simulink model "SF102A_MotCtrlPrmEstimn"  (R2013b)
settings: Solver=FixedStepDiscrete  StartTime=0.0  StopTime=1  FixedStep=0.002  RelTol=1e-3
values from neighbouring files (symbols this model uses):
  MotCtrlPrmEstimnFetRNom = DataDict.Calibration    [SF102A_MotCtrlPrmEstimn_DataDict.m]
  MotCtrlPrmEstimnFetThermCoeff = DataDict.Calibration    [SF102A_MotCtrlPrmEstimn_DataDict.m]
  MotCtrlPrmEstimnMagThermCoeff = DataDict.Calibration    [SF102A_MotCtrlPrmEstimn_DataDict.m]
  MotCtrlPrmEstimnMotBackEmfConNom = DataDict.Calibration    [SF102A_MotCtrlPrmEstimn_DataDict.m]
  MotCtrlPrmEstimnMotBackEmfConSatnScaIvtrLoaMtgtn = DataDict.Calibration    [SF102A_MotCtrlPrmEstimn_DataDict.m]
  MotCtrlPrmEstimnMotInduDaxIvtrLoaMtgtn = DataDict.Calibration    [SF102A_MotCtrlPrmEstimn_DataDict.m]
  MotCtrlPrmEstimnMotInduDaxNom = DataDict.Calibration    [SF102A_MotCtrlPrmEstimn_DataDict.m]
  MotCtrlPrmEstimnMotInduQaxIvtrLoaMtgtn = DataDict.Calibration    [SF102A_MotCtrlPrmEstimn_DataDict.m]
  MotCtrlPrmEstimnMotInduQaxNom = DataDict.Calibration    [SF102A_MotCtrlPrmEstimn_DataDict.m]
  MotCtrlPrmEstimnMotRNom = DataDict.Calibration    [SF102A_MotCtrlPrmEstimn_DataDict.m]
  MotCtrlPrmEstimnMotWidgThermCoeff = DataDict.Calibration    [SF102A_MotCtrlPrmEstimn_DataDict.m]
  MotCtrlPrmEstimnTNom = DataDict.Calibration    [SF102A_MotCtrlPrmEstimn_DataDict.m]
libraries: NxtrLim x12, NxtrNvM x3, FixdToFloat x3, FloatToFixd x2, BilnrIntrpnCmnX x2, simulink x1, LnrIntrpn x1
(part 2 of 2)

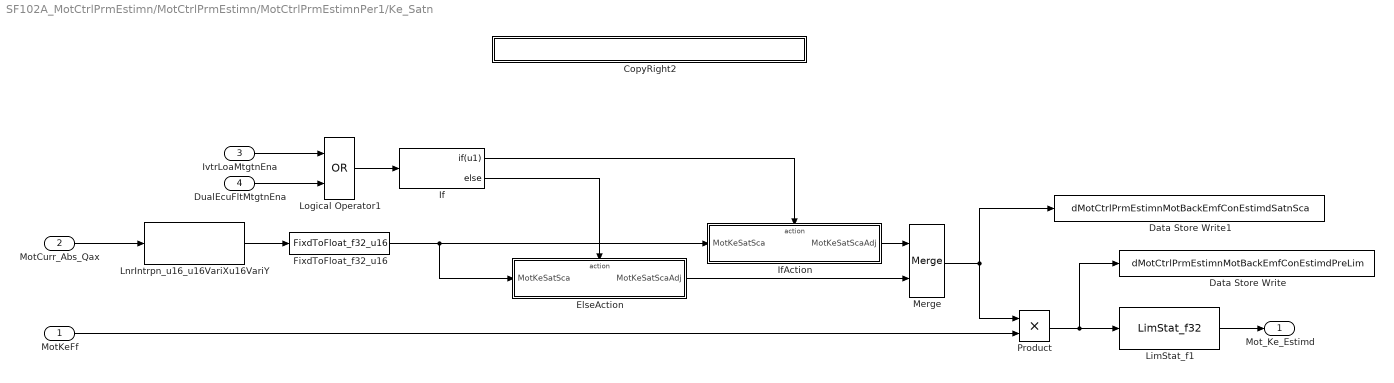
== system SF102A_MotCtrlPrmEstimn/MotCtrlPrmEstimn/MotCtrlPrmEstimnPer1/Ke_Satn ==
  MotKeFf : Inport  RequirementInfo="{'linktype_rmi_doors' '0000bb41 (/E-STEER Core/SubSystem Specifications/Application Functions/SF99/SF102A Motor Control Parameter Estimation)' '#SF102A_51' 'true' 'REQ:  SF102A_51' '' } %GIDa_ca68ec69_3fc5_4f7c_b88c_595812cbfbcb"
  MotCurr_Abs_Qax : Inport  RequirementInfo="{'linktype_rmi_doors' '0000bb41 (/E-STEER Core/SubSystem Specifications/Application Functions/SF99/SF102A Motor Control Parameter Estimation)' '#SF102A_50' 'true' 'REQ:  SF102A_50' '' ; 'linktype_rmi_doors' '0000bb41 (/E-STEER Core/SubSystem Specifications/Application Functions/SF99/SF102A Motor Control Parameter Estimation)' '#SF102A_51' 'true' 'REQ:  SF102A_51' '' } %GIDa_2c278c4c_34d3_4811_86bc_36d03b3a96ac"  Port=2
  IvtrLoaMtgtnEna : Inport  RequirementInfo={} %GIDa_55b474c1_2280_46dc_85c4_036e6c47f197  Port=3
  DualEcuFltMtgtnEna : Inport  RequirementInfo={} %GIDa_d4aecfc1_0bde_4cba_a1f2_c868140dd92f  Port=4
  CopyRight2 : Subsystem  Description=|  mask(Copyright Information){none=on}
      | Copyright info block.                                               
      |                                                                     
      | Place copyright information at the top of every subsystem in design.
      mask prompts: none "No parameters"
      mask help: Place copyright information at the top of every subsystem in design.
      mask Display:
      | NxtrConf = 'Nexteer Confidential';
      | 
      | sys = bdroot; %handle for the current model ("system")
      | first = get_param(sys,'Created');
      | if(isempty(first))
      |     first = datestr(now,'yyyy');
      | else
      |     first = first(end-3:end);  %year is last four digits
      | end
      | 
      | last = get_param(sys,'LastModifiedDate');
      | if isempty(last)
      |     last = datestr(now,'yyyy');
      | else
      |     last = last(end-3:end);
      | end
      | 
      | if strcmp(first,last)
      |     fprintf('%s -- Copyright %s Nexteer',NxtrConf,first)
      | else
      |     fprintf('%s -- %s%s- %s Nexteer',NxtrConf,char(169),first,last)
      | end
  Data Store Write : DataStoreWrite  DataStoreName=dMotCtrlPrmEstimnMotBackEmfConEstimdPreLim
  Data Store Write1 : DataStoreWrite  DataStoreName=dMotCtrlPrmEstimnMotBackEmfConEstimdSatnSca
  ElseAction : Subsystem  RequirementInfo={'linktype_rmi_doors' '0000bb41 (/E-STEER Core/SubSystem Specifications/Application Functions/SF99/SF102A Motor Control Parameter Estimation)' '#SF102A_98' 'true' 'REQ:SF102A_98' '' } %GIDa_66276068_9c00_412a_ba6b_6416dc8d8b98  TreatAsAtomicUnit=on
  FixdToFloat_f32_u16 : FixdToFloat/FixdToFloat_f32_u16  RequirementInfo="{'linktype_rmi_doors' '0000bb41 (/E-STEER Core/SubSystem Specifications/Application Functions/SF99/SF102A Motor Control Parameter Estimation)' '#SF102A_50' 'true' 'REQ:  SF102A_50' '' ; 'linktype_rmi_doors' '0000bb41 (/E-STEER Core/SubSystem Specifications/Application Functions/SF99/SF102A Motor Control Parameter Estimation)' '#SF102A_51' 'true' 'REQ:  SF102A_51' '' } %GIDa_30ff50c8_3b22_4b0c_a269_05ad7e058210"  Param1=14
  If : If  RequirementInfo={'linktype_rmi_doors' '0000bb41 (/E-STEER Core/SubSystem Specifications/Application Functions/SF99/SF102A Motor Control Parameter Estimation)' '#SF102A_98' 'true' 'REQ:SF102A_98' '' } %GIDa_a3456abc_87ca_4b4f_a759_32778ebeb971  IfExpression=u1
  IfAction : Subsystem  RequirementInfo={'linktype_rmi_doors' '0000bb41 (/E-STEER Core/SubSystem Specifications/Application Functions/SF99/SF102A Motor Control Parameter Estimation)' '#SF102A_98' 'true' 'REQ:SF102A_98' '' } %GIDa_37ca894a_f849_476d_86bb_7b83343cfe71  TreatAsAtomicUnit=on
      settings: RTWSystemCode=Inline
  LimStat_f1 : NxtrLim/LimStat_f32  RequirementInfo="{'linktype_rmi_doors' '0000bb41 (/E-STEER Core/SubSystem Specifications/Application Functions/SF99/SF102A Motor Control Parameter Estimation)' '#SF102A_58' 'true' 'REQ:  SF102A_58' '' ; 'linktype_rmi_doors' '0000bb41 (/E-STEER Core/SubSystem Specifications/Application Functions/SF99/SF102A Motor Control Parameter Estimation)' '#SF102A_77' 'true' 'REQ:  SF102A_77' '' } %GIDa_efba97fb_19df_4fbb_835b_1b2e4b8dafc6"  LoLim=MotCtrlPrmEstimnMotBackEmfConLoLim  HiLim=MotCtrlPrmEstimnMotBackEmfConHiLim
      settings: AttributesFormatString=|
      | Low Limit: %<LoLim>
      | High Limit:%<HiLim>
  LnrIntrpn_u16_u16VariXu16VariY : LnrIntrpn/LnrIntrpn_u16_u16VariXu16VariY  RequirementInfo="{'linktype_rmi_doors' '0000bb41 (/E-STEER Core/SubSystem Specifications/Application Functions/SF99/SF102A Motor Control Parameter Estimation)' '#SF102A_50' 'true' 'REQ:  SF102A_50' '' ; 'linktype_rmi_doors' '0000bb41 (/E-STEER Core/SubSystem Specifications/Application Functions/SF99/SF102A Motor Control Parameter Estimation)' '#SF102A_51' 'true' 'REQ:  SF102A_51' '' } %GIDa_d0625b03_476d_4e45_a255_0ebee113fbee"  XTbl=MotCtrlPrmEstimnMotBackEmfConSatnX  YTbl=MotCtrlPrmEstimnMotBackEmfConSatnY
      settings: AttributesFormatString=Lnr ( u16VariX , u16VariY )
  Logical Operator1 : Logic  Operator=OR  AllPortsSameDT=off  OutDataTypeStr=boolean
  Merge : Merge  RequirementInfo={'linktype_rmi_doors' '0000bb41 (/E-STEER Core/SubSystem Specifications/Application Functions/SF99/SF102A Motor Control Parameter Estimation)' '#SF102A_98' 'true' 'REQ:SF102A_98' '' } %GIDa_a953d2b4_b957_47a9_9e6b_14a5c79d3b44
  Product : Product  RequirementInfo="{'linktype_rmi_doors' '0000bb41 (/E-STEER Core/SubSystem Specifications/Application Functions/SF99/SF102A Motor Control Parameter Estimation)' '#SF102A_51' 'true' 'REQ:  SF102A_51' '' } %GIDa_5f6ae74a_60fe_41e9_b3da_6065efd4cb7b"
  Mot_Ke_Estimd : Outport  RequirementInfo="{'linktype_rmi_doors' '0000bb41 (/E-STEER Core/SubSystem Specifications/Application Functions/SF99/SF102A Motor Control Parameter Estimation)' '#SF102A_51' 'true' 'REQ:  SF102A_51' '' } %GIDa_09a11d9d_3369_4bbb_9775_2492efeb312e"
  wires:
  LnrIntrpn_u16_u16VariXu16VariY/1 -> FixdToFloat_f32_u16/1
  MotKeFf/1 -> Product/2
  Product/1 -> Data Store Write/1, LimStat_f1/1
  LimStat_f1/1 -> Mot_Ke_Estimd/1
  Merge/1 -> Product/1, Data Store Write1/1
  MotCurr_Abs_Qax/1 -> LnrIntrpn_u16_u16VariXu16VariY/1
  If/2 -> ElseAction/Action
  If/1 -> IfAction/Action
  ElseAction/1(MotKeSatScaAdj) -> Merge/2
  IfAction/1(MotKeSatScaAdj) -> Merge/1
  FixdToFloat_f32_u16/1 -> ElseAction/1(MotKeSatSca), IfAction/1(MotKeSatSca)
  IvtrLoaMtgtnEna/1 -> Logical Operator1/1
  DualEcuFltMtgtnEna/1 -> Logical Operator1/2
  Logical Operator1/1 -> If/1

== system SF102A_MotCtrlPrmEstimn/MotCtrlPrmEstimn/MotCtrlPrmEstimnPer2/CopyRight2 ==

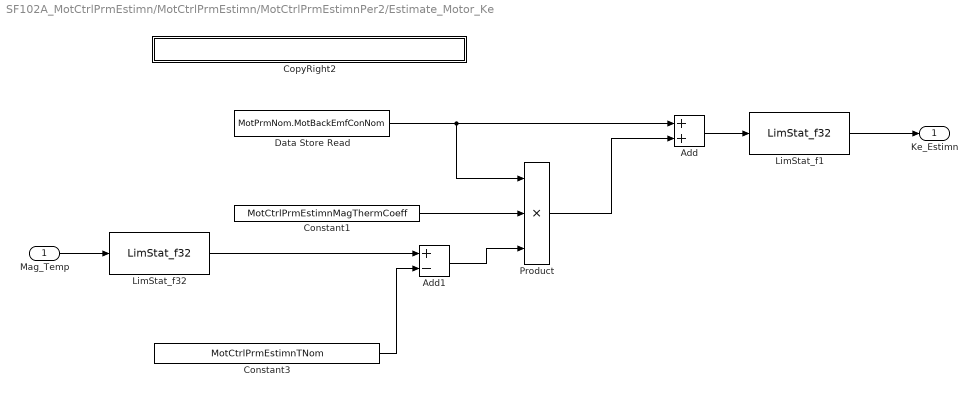
== system SF102A_MotCtrlPrmEstimn/MotCtrlPrmEstimn/MotCtrlPrmEstimnPer2/Estimate_Motor_Ke ==
  Mag_Temp : Inport  RequirementInfo="{'linktype_rmi_doors' '0000bb41 (/E-STEER Core/SubSystem Specifications/Application Functions/SF99/SF102A Motor Control Parameter Estimation)' '#SF102A_79' 'true' 'REQ:  SF102A_79' '' } %GIDa_27ec31af_a9b0_49cc_af07_57667b1f493e"
  Add : Sum  RequirementInfo="{'linktype_rmi_doors' '0000bb41 (/E-STEER Core/SubSystem Specifications/Application Functions/SF99/SF102A Motor Control Parameter Estimation)' '#SF102A_79' 'true' 'REQ:  SF102A_79' '' } %GIDa_032c7cc2_7709_47c2_b088_cd2d10e989b2"
  Add1 : Sum  RequirementInfo="{'linktype_rmi_doors' '0000bb41 (/E-STEER Core/SubSystem Specifications/Application Functions/SF99/SF102A Motor Control Parameter Estimation)' '#SF102A_79' 'true' 'REQ:  SF102A_79' '' } %GIDa_325acd5b_255d_4854_912c_df54e826c433"  Inputs=+-
  Constant1 : Constant  RequirementInfo="{'linktype_rmi_doors' '0000bb41 (/E-STEER Core/SubSystem Specifications/Application Functions/SF99/SF102A Motor Control Parameter Estimation)' '#SF102A_79' 'true' 'REQ:  SF102A_79' '' } %GIDa_95a68016_cdb7_4865_bd2d_230faec756a9"  Value=MotCtrlPrmEstimnMagThermCoeff
  Constant3 : Constant  RequirementInfo="{'linktype_rmi_doors' '0000bb41 (/E-STEER Core/SubSystem Specifications/Application Functions/SF99/SF102A Motor Control Parameter Estimation)' '#SF102A_79' 'true' 'REQ:  SF102A_79' '' } %GIDa_62d1b4b8_0c50_4cfb_896c_98b14855d1cc"  Value=MotCtrlPrmEstimnTNom
  CopyRight2 : Subsystem  Description=|  mask(Copyright Information){none=on}
      | Copyright info block.                                               
      |                                                                     
      | Place copyright information at the top of every subsystem in design.
      mask prompts: none "No parameters"
      mask help: Place copyright information at the top of every subsystem in design.
      mask Display:
      | NxtrConf = 'Nexteer Confidential';
      | 
      | sys = bdroot; %handle for the current model ("system")
      | first = get_param(sys,'Created');
      | if(isempty(first))
      |     first = datestr(now,'yyyy');
      | else
      |     first = first(end-3:end);  %year is last four digits
      | end
      | 
      | last = get_param(sys,'LastModifiedDate');
      | if isempty(last)
      |     last = datestr(now,'yyyy');
      | else
      |     last = last(end-3:end);
      | end
      | 
      | if strcmp(first,last)
      |     fprintf('%s -- Copyright %s Nexteer',NxtrConf,first)
      | else
      |     fprintf('%s -- %s%s- %s Nexteer',NxtrConf,char(169),first,last)
      | end
  Data Store Read : DataStoreRead  RequirementInfo="{'linktype_rmi_doors' '0000bb41 (/E-STEER Core/SubSystem Specifications/Application Functions/SF99/SF102A Motor Control Parameter Estimation)' '#SF102A_79' 'true' 'REQ:  SF102A_79' '' } %GIDa_645f74b9_1f8d_46ad_9bf2_de69bb92e4a8"  DataStoreName=MotPrmNom  DataStoreElements=MotPrmNom.MotBackEmfConNom
  LimStat_f1 : NxtrLim/LimStat_f32  RequirementInfo="{'linktype_rmi_doors' '0000bb41 (/E-STEER Core/SubSystem Specifications/Application Functions/SF99/SF102A Motor Control Parameter Estimation)' '#SF102A_58' 'true' 'REQ:  SF102A_58' '' ; 'linktype_rmi_doors' '0000bb41 (/E-STEER Core/SubSystem Specifications/Application Functions/SF99/SF102A Motor Control Parameter Estimation)' '#SF102A_77' 'true' 'REQ:  SF102A_77' '' } %GIDa_eaf1ef11_d061_4c62_ac0d_c6cc858486f6"  LoLim=MotCtrlPrmEstimnMotBackEmfConLoLim  HiLim=MotCtrlPrmEstimnMotBackEmfConHiLim
      settings: AttributesFormatString=|
      | Low Limit: %<LoLim>
      | High Limit:%<HiLim>
  LimStat_f32 : NxtrLim/LimStat_f32  RequirementInfo="{'linktype_rmi_doors' '0000bb41 (/E-STEER Core/SubSystem Specifications/Application Functions/SF99/SF102A Motor Control Parameter Estimation)' '#SF102A_79' 'true' 'REQ:  SF102A_79' '' ; 'linktype_rmi_doors' '0000bb41 (/E-STEER Core/SubSystem Specifications/Application Functions/SF99/SF102A Motor Control Parameter Estimation)' '#SF102A_77' 'true' 'REQ:  SF102A_77' '' ; 'linktype_rmi_doors' '0000bb41 (/E-STEER Core/SubSystem Specifications/Application Functions/SF99/SF102A Motor Control Parameter Estimation)' '#SF102A_78' 'true' 'REQ:  SF102A_78' '' } %GIDa_c2f1950b_3da8_40ec_be6a_a30c98ab318e"  LoLim=MAGNETTESTLOLIM_DEGCGRD_F32  HiLim=MAGNETTESTHILIM_DEGCGRD_F32
      settings: AttributesFormatString=|
      | Low Limit: %<LoLim>
      | High Limit:%<HiLim>
  Product : Product  RequirementInfo="{'linktype_rmi_doors' '0000bb41 (/E-STEER Core/SubSystem Specifications/Application Functions/SF99/SF102A Motor Control Parameter Estimation)' '#SF102A_79' 'true' 'REQ:  SF102A_79' '' } %GIDa_beae5c53_6cdc_4a5b_91cf_3f5121611092"  Inputs=3
  Ke_Estimn : Outport  RequirementInfo="{'linktype_rmi_doors' '0000bb41 (/E-STEER Core/SubSystem Specifications/Application Functions/SF99/SF102A Motor Control Parameter Estimation)' '#SF102A_79' 'true' 'REQ:  SF102A_79' '' } %GIDa_fc83a985_17ec_4189_8e4e_4c54ef9d1b52"
  wires:
  Data Store Read/1 -> Add/1, Product/1
  Mag_Temp/1 -> LimStat_f32/1
  Constant3/1 -> Add1/2
  Add1/1 -> Product/3
  Constant1/1 -> Product/2
  Product/1 -> Add/2
  LimStat_f32/1 -> Add1/1
  Add/1 -> LimStat_f1/1
  LimStat_f1/1 -> Ke_Estimn/1

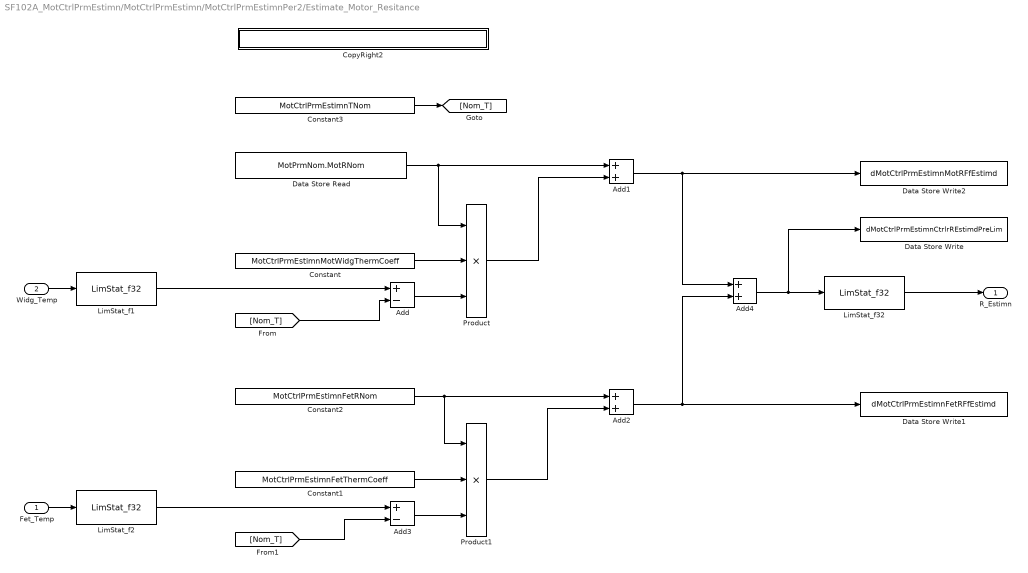
== system SF102A_MotCtrlPrmEstimn/MotCtrlPrmEstimn/MotCtrlPrmEstimnPer2/Estimate_Motor_Resitance ==
  Fet_Temp : Inport  RequirementInfo="{'linktype_rmi_doors' '0000bb41 (/E-STEER Core/SubSystem Specifications/Application Functions/SF99/SF102A Motor Control Parameter Estimation)' '#SF102A_79' 'true' 'REQ:  SF102A_79' '' } %GIDa_71261e82_d55a_46e2_88a5_a0108b8fb2d0"
  Widg_Temp : Inport  RequirementInfo="{'linktype_rmi_doors' '0000bb41 (/E-STEER Core/SubSystem Specifications/Application Functions/SF99/SF102A Motor Control Parameter Estimation)' '#SF102A_79' 'true' 'REQ:  SF102A_79' '' } %GIDa_114d5c54_a76c_45b6_89e5_6083f63a86c5"  Port=2
  Add : Sum  RequirementInfo="{'linktype_rmi_doors' '0000bb41 (/E-STEER Core/SubSystem Specifications/Application Functions/SF99/SF102A Motor Control Parameter Estimation)' '#SF102A_79' 'true' 'REQ:  SF102A_79' '' } %GIDa_9b0531e8_817d_417f_b08e_d44cb601da31"  Inputs=+-
  Add1 : Sum  RequirementInfo="{'linktype_rmi_doors' '0000bb41 (/E-STEER Core/SubSystem Specifications/Application Functions/SF99/SF102A Motor Control Parameter Estimation)' '#SF102A_79' 'true' 'REQ:  SF102A_79' '' } %GIDa_233736cd_2ef7_40b2_bc6f_cb61d0fd07dc"
  Add2 : Sum  RequirementInfo="{'linktype_rmi_doors' '0000bb41 (/E-STEER Core/SubSystem Specifications/Application Functions/SF99/SF102A Motor Control Parameter Estimation)' '#SF102A_79' 'true' 'REQ:  SF102A_79' '' } %GIDa_91af04b1_221a_42c8_9042_f241f3590e10"
  Add3 : Sum  RequirementInfo="{'linktype_rmi_doors' '0000bb41 (/E-STEER Core/SubSystem Specifications/Application Functions/SF99/SF102A Motor Control Parameter Estimation)' '#SF102A_79' 'true' 'REQ:  SF102A_79' '' } %GIDa_3a49abd4_5a0a_43ef_a101_a021352c1f05"  Inputs=+-
  Add4 : Sum  RequirementInfo="{'linktype_rmi_doors' '0000bb41 (/E-STEER Core/SubSystem Specifications/Application Functions/SF99/SF102A Motor Control Parameter Estimation)' '#SF102A_79' 'true' 'REQ:  SF102A_79' '' ; 'linktype_rmi_doors' '0000bb41 (/E-STEER Core/SubSystem Specifications/Application Functions/SF99/SF102A Motor Control Parameter Estimation)' '#SF102A_80' 'true' 'REQ:  SF102A_80' '' } %GIDa_9a8c8a44_bb52_4b56_826d_532e182878d7"
  Constant : Constant  RequirementInfo="{'linktype_rmi_doors' '0000bb41 (/E-STEER Core/SubSystem Specifications/Application Functions/SF99/SF102A Motor Control Parameter Estimation)' '#SF102A_79' 'true' 'REQ:  SF102A_79' '' } %GIDa_9b025c1a_f7a9_4777_8ff0_3314b9890bfc"  Value=MotCtrlPrmEstimnMotWidgThermCoeff
  Constant1 : Constant  RequirementInfo="{'linktype_rmi_doors' '0000bb41 (/E-STEER Core/SubSystem Specifications/Application Functions/SF99/SF102A Motor Control Parameter Estimation)' '#SF102A_79' 'true' 'REQ:  SF102A_79' '' } %GIDa_6745513d_e9f0_42ff_93c4_399939918044"  Value=MotCtrlPrmEstimnFetThermCoeff
  Constant2 : Constant  RequirementInfo="{'linktype_rmi_doors' '0000bb41 (/E-STEER Core/SubSystem Specifications/Application Functions/SF99/SF102A Motor Control Parameter Estimation)' '#SF102A_79' 'true' 'REQ:  SF102A_79' '' } %GIDa_eba00650_623e_448f_ba0b_e87ab14d84b4"  Value=MotCtrlPrmEstimnFetRNom
  Constant3 : Constant  RequirementInfo="{'linktype_rmi_doors' '0000bb41 (/E-STEER Core/SubSystem Specifications/Application Functions/SF99/SF102A Motor Control Parameter Estimation)' '#SF102A_79' 'true' 'REQ:  SF102A_79' '' } %GIDa_0212b6ce_dff5_41d0_8898_d0ec0ff62430"  Value=MotCtrlPrmEstimnTNom
  CopyRight2 : Subsystem  Description=|  mask(Copyright Information){none=on}
      | Copyright info block.                                               
      |                                                                     
      | Place copyright information at the top of every subsystem in design.
      mask prompts: none "No parameters"
      mask help: Place copyright information at the top of every subsystem in design.
      mask Display:
      | NxtrConf = 'Nexteer Confidential';
      | 
      | sys = bdroot; %handle for the current model ("system")
      | first = get_param(sys,'Created');
      | if(isempty(first))
      |     first = datestr(now,'yyyy');
      | else
      |     first = first(end-3:end);  %year is last four digits
      | end
      | 
      | last = get_param(sys,'LastModifiedDate');
      | if isempty(last)
      |     last = datestr(now,'yyyy');
      | else
      |     last = last(end-3:end);
      | end
      | 
      | if strcmp(first,last)
      |     fprintf('%s -- Copyright %s Nexteer',NxtrConf,first)
      | else
      |     fprintf('%s -- %s%s- %s Nexteer',NxtrConf,char(169),first,last)
      | end
  Data Store Read : DataStoreRead  RequirementInfo="{'linktype_rmi_doors' '0000bb41 (/E-STEER Core/SubSystem Specifications/Application Functions/SF99/SF102A Motor Control Parameter Estimation)' '#SF102A_79' 'true' 'REQ:  SF102A_79' '' } %GIDa_7acda2c8_c589_429d_b3c9_76fb565b8f54"  DataStoreName=MotPrmNom  DataStoreElements=MotPrmNom.MotRNom
  Data Store Write : DataStoreWrite  RequirementInfo="{'linktype_rmi_doors' '0000bb41 (/E-STEER Core/SubSystem Specifications/Application Functions/SF99/SF102A Motor Control Parameter Estimation)' '#SF102A_79' 'true' 'REQ:  SF102A_79' '' } %GIDa_bc42402b_ab84_4d6d_9d03_69266616b3e8"  DataStoreName=dMotCtrlPrmEstimnCtrlrREstimdPreLim
  Data Store Write1 : DataStoreWrite  RequirementInfo="{'linktype_rmi_doors' '0000bb41 (/E-STEER Core/SubSystem Specifications/Application Functions/SF99/SF102A Motor Control Parameter Estimation)' '#SF102A_79' 'true' 'REQ:  SF102A_79' '' } %GIDa_36430a93_3b27_413d_b072_2176415a3790"  DataStoreName=dMotCtrlPrmEstimnFetRFfEstimd
  Data Store Write2 : DataStoreWrite  RequirementInfo="{'linktype_rmi_doors' '0000bb41 (/E-STEER Core/SubSystem Specifications/Application Functions/SF99/SF102A Motor Control Parameter Estimation)' '#SF102A_79' 'true' 'REQ:  SF102A_79' '' } %GIDa_80c5e666_2473_42f1_86ef_82fc80078736"  DataStoreName=dMotCtrlPrmEstimnMotRFfEstimd
  LimStat_f1 : NxtrLim/LimStat_f32  RequirementInfo="{'linktype_rmi_doors' '0000bb41 (/E-STEER Core/SubSystem Specifications/Application Functions/SF99/SF102A Motor Control Parameter Estimation)' '#SF102A_79' 'true' 'REQ:  SF102A_79' '' ; 'linktype_rmi_doors' '0000bb41 (/E-STEER Core/SubSystem Specifications/Application Functions/SF99/SF102A Motor Control Parameter Estimation)' '#SF102A_77' 'true' 'REQ:  SF102A_77' '' ; 'linktype_rmi_doors' '0000bb41 (/E-STEER Core/SubSystem Specifications/Application Functions/SF99/SF102A Motor Control Parameter Estimation)' '#SF102A_78' 'true' 'REQ:  SF102A_78' '' } %GIDa_fb3a749c_4275_4f33_aff8_cacb0d673586"  LoLim=MOTWIDGTESTLOLIM_DEGCGRD_F32  HiLim=MOTWIDGTESTHILIM_DEGCGRD_F32
      settings: AttributesFormatString=|
      | Low Limit: %<LoLim>
      | High Limit:%<HiLim>
  LimStat_f2 : NxtrLim/LimStat_f32  RequirementInfo="{'linktype_rmi_doors' '0000bb41 (/E-STEER Core/SubSystem Specifications/Application Functions/SF99/SF102A Motor Control Parameter Estimation)' '#SF102A_79' 'true' 'REQ:  SF102A_79' '' ; 'linktype_rmi_doors' '0000bb41 (/E-STEER Core/SubSystem Specifications/Application Functions/SF99/SF102A Motor Control Parameter Estimation)' '#SF102A_77' 'true' 'REQ:  SF102A_77' '' ; 'linktype_rmi_doors' '0000bb41 (/E-STEER Core/SubSystem Specifications/Application Functions/SF99/SF102A Motor Control Parameter Estimation)' '#SF102A_78' 'true' 'REQ:  SF102A_78' '' } %GIDa_14098e71_f3b2_499e_9663_4f83a83d48b1"  LoLim=FETTESTLOLIM_DEGCGRD_F32  HiLim=FETTESTHILIM_DEGCGRD_F32
      settings: AttributesFormatString=|
      | Low Limit: %<LoLim>
      | High Limit:%<HiLim>
  LimStat_f32 : NxtrLim/LimStat_f32  RequirementInfo="{'linktype_rmi_doors' '0000bb41 (/E-STEER Core/SubSystem Specifications/Application Functions/SF99/SF102A Motor Control Parameter Estimation)' '#SF102A_59' 'true' 'REQ:  SF102A_59' '' ; 'linktype_rmi_doors' '0000bb41 (/E-STEER Core/SubSystem Specifications/Application Functions/SF99/SF102A Motor Control Parameter Estimation)' '#SF102A_77' 'true' 'REQ:  SF102A_77' '' } %GIDa_89ba3e5e_07f1_4c82_82e6_4d27441737fa"  LoLim=MotCtrlPrmEstimnMotRLoLim  HiLim=MotCtrlPrmEstimnMotRHiLim
      settings: AttributesFormatString=|
      | Low Limit: %<LoLim>
      | High Limit:%<HiLim>
  Product : Product  RequirementInfo="{'linktype_rmi_doors' '0000bb41 (/E-STEER Core/SubSystem Specifications/Application Functions/SF99/SF102A Motor Control Parameter Estimation)' '#SF102A_79' 'true' 'REQ:  SF102A_79' '' } %GIDa_af4e4b3b_5491_4068_93d0_bb891534fbdf"  Inputs=3
  Product1 : Product  RequirementInfo="{'linktype_rmi_doors' '0000bb41 (/E-STEER Core/SubSystem Specifications/Application Functions/SF99/SF102A Motor Control Parameter Estimation)' '#SF102A_79' 'true' 'REQ:  SF102A_79' '' } %GIDa_d5f5b513_6bb5_476e_8ea9_0a7eb453636c"  Inputs=3
  R_Estimn : Outport  RequirementInfo="{'linktype_rmi_doors' '0000bb41 (/E-STEER Core/SubSystem Specifications/Application Functions/SF99/SF102A Motor Control Parameter Estimation)' '#SF102A_79' 'true' 'REQ:  SF102A_79' '' } %GIDa_f8f6770c_7aa5_474b_b987_cea594cab94f"
  wires:
  LimStat_f32/1 -> R_Estimn/1
  Add/1 -> Product/3
  Widg_Temp/1 -> LimStat_f1/1
  Constant3/1 -> [Nom_T]
  [Nom_T] -> Add/2
  Data Store Read/1 -> Product/1, Add1/1
  Constant/1 -> Product/2
  Product/1 -> Add1/2
  Constant2/1 -> Add2/1, Product1/1
  Product1/1 -> Add2/2
  Constant1/1 -> Product1/2
  Add3/1 -> Product1/3
  Add2/1 -> Data Store Write1/1, Add4/2
  Add4/1 -> Data Store Write/1, LimStat_f32/1
  Fet_Temp/1 -> LimStat_f2/1
  [Nom_T] -> Add3/2
  LimStat_f1/1 -> Add/1
  LimStat_f2/1 -> Add3/1
  Add1/1 -> Data Store Write2/1, Add4/1

== system SF102A_MotCtrlPrmEstimn/MotCtrlPrmEstimn/SetMotPrmNomEol/CopyRight2 ==

== system SF102A_MotCtrlPrmEstimn/MotCtrlPrmEstimn/MotCtrlPrmEstimnInit1/NVM is NOT okay/CopyRight2 ==

== system SF102A_MotCtrlPrmEstimn/MotCtrlPrmEstimn/MotCtrlPrmEstimnInit1/NVM is okay/CopyRight2 ==

== system SF102A_MotCtrlPrmEstimn/MotCtrlPrmEstimn/MotCtrlPrmEstimnPer1/Indu_Satn/CopyRight2 ==

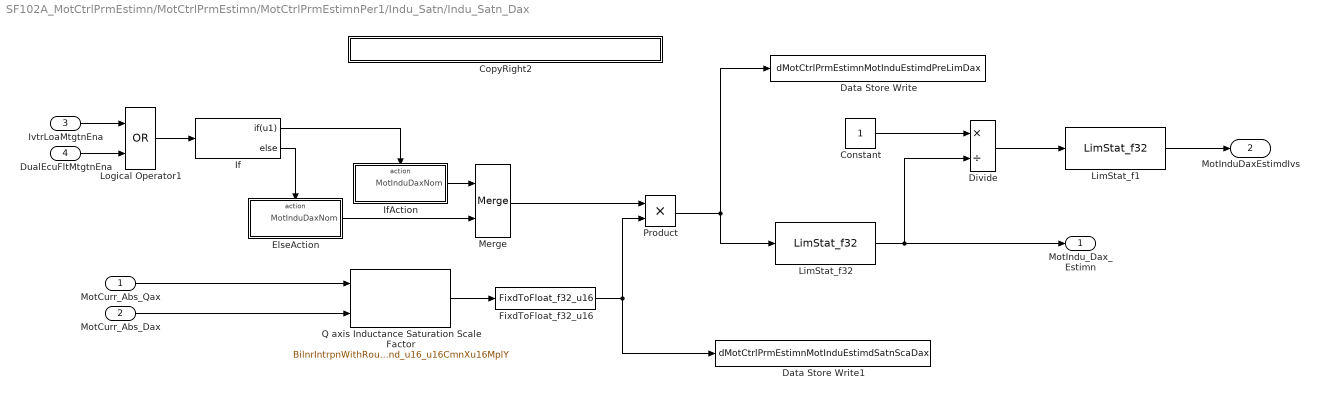
== system SF102A_MotCtrlPrmEstimn/MotCtrlPrmEstimn/MotCtrlPrmEstimnPer1/Indu_Satn/Indu_Satn_Dax ==
  MotCurr_Abs_Qax : Inport  RequirementInfo="{'linktype_rmi_doors' '0000bb41 (/E-STEER Core/SubSystem Specifications/Application Functions/SF99/SF102A Motor Control Parameter Estimation)' '#SF102A_56' 'true' 'REQ:  SF102A_56' '' ; 'linktype_rmi_doors' '0000bb41 (/E-STEER Core/SubSystem Specifications/Application Functions/SF99/SF102A Motor Control Parameter Estimation)' '#SF102A_55' 'true' 'REQ:  SF102A_55' '' } %GIDa_ef40171d_4779_48df_9fac_07718011ef63"
  MotCurr_Abs_Dax : Inport  RequirementInfo="{'linktype_rmi_doors' '0000bb41 (/E-STEER Core/SubSystem Specifications/Application Functions/SF99/SF102A Motor Control Parameter Estimation)' '#SF102A_56' 'true' 'REQ:  SF102A_56' '' ; 'linktype_rmi_doors' '0000bb41 (/E-STEER Core/SubSystem Specifications/Application Functions/SF99/SF102A Motor Control Parameter Estimation)' '#SF102A_55' 'true' 'REQ:  SF102A_55' '' } %GIDa_5cd76948_db79_46f9_bc8c_9d5690763c26"  Port=2
  IvtrLoaMtgtnEna : Inport  RequirementInfo={} %GIDa_8f7f0911_4fea_4dc1_9951_6685daf7156c  Port=3
  DualEcuFltMtgtnEna : Inport  RequirementInfo={} %GIDa_1e00389d_d1a3_48ef_a0bf_5c839fd5079d  Port=4
  Constant : Constant  RequirementInfo={} %GIDa_2e9a586d_d80b_42bf_b653_0d9ac14fbba9  OutDataTypeStr=single
  CopyRight2 : Subsystem  Description=|  mask(Copyright Information){none=on}
      | Copyright info block.                                               
      |                                                                     
      | Place copyright information at the top of every subsystem in design.
      mask prompts: none "No parameters"
      mask help: Place copyright information at the top of every subsystem in design.
      mask Display:
      | NxtrConf = 'Nexteer Confidential';
      | 
      | sys = bdroot; %handle for the current model ("system")
      | first = get_param(sys,'Created');
      | if(isempty(first))
      |     first = datestr(now,'yyyy');
      | else
      |     first = first(end-3:end);  %year is last four digits
      | end
      | 
      | last = get_param(sys,'LastModifiedDate');
      | if isempty(last)
      |     last = datestr(now,'yyyy');
      | else
      |     last = last(end-3:end);
      | end
      | 
      | if strcmp(first,last)
      |     fprintf('%s -- Copyright %s Nexteer',NxtrConf,first)
      | else
      |     fprintf('%s -- %s%s- %s Nexteer',NxtrConf,char(169),first,last)
      | end
  Data Store Write : DataStoreWrite  DataStoreName=dMotCtrlPrmEstimnMotInduEstimdPreLimDax
  Data Store Write1 : DataStoreWrite  DataStoreName=dMotCtrlPrmEstimnMotInduEstimdSatnScaDax
  Divide : Product  Inputs=*/
  ElseAction : Subsystem  RequirementInfo={'linktype_rmi_doors' '0000bb41 (/E-STEER Core/SubSystem Specifications/Application Functions/SF99/SF102A Motor Control Parameter Estimation)' '#SF102A_92' 'true' 'REQ:SF102A_92' '' } %GIDa_4b50fb5b_4140_4633_a9b2_a86424d84563  TreatAsAtomicUnit=on
  FixdToFloat_f32_u16 : FixdToFloat/FixdToFloat_f32_u16  RequirementInfo="{'linktype_rmi_doors' '0000bb41 (/E-STEER Core/SubSystem Specifications/Application Functions/SF99/SF102A Motor Control Parameter Estimation)' '#SF102A_56' 'true' 'REQ:  SF102A_56' '' } %GIDa_9a95dfbb_30b3_4b7d_828f_0516f9c31278"  Param1=14
  If : If  RequirementInfo={'linktype_rmi_doors' '0000bb41 (/E-STEER Core/SubSystem Specifications/Application Functions/SF99/SF102A Motor Control Parameter Estimation)' '#SF102A_92' 'true' 'REQ:SF102A_92' '' } %GIDa_3f34e804_2849_47ef_b731_de68500adcf3  IfExpression=u1
  IfAction : Subsystem  RequirementInfo={'linktype_rmi_doors' '0000bb41 (/E-STEER Core/SubSystem Specifications/Application Functions/SF99/SF102A Motor Control Parameter Estimation)' '#SF102A_92' 'true' 'REQ:SF102A_92' '' } %GIDa_ce7dbb5f_bb89_4e61_ae36_5b1a6b5cebf7  TreatAsAtomicUnit=on
      settings: RTWSystemCode=Inline
  LimStat_f1 : NxtrLim/LimStat_f32  RequirementInfo="{'linktype_rmi_doors' '0000bb41 (/E-STEER Core/SubSystem Specifications/Application Functions/SF99/SF102A Motor Control Parameter Estimation)' '#SF102A_77' 'true' 'REQ:  SF102A_77' '' } %GIDa_89d990b6_7ecb_4be9_9002_643b2b633094"  LoLim=MOTINDUIVSLOLIM_IVSHENRY_F32  HiLim=MOTINDUIVSHILIM_IVSHENRY_F32
      settings: AttributesFormatString=|
      | Low Limit: %<LoLim>
      | High Limit:%<HiLim>
  LimStat_f32 : NxtrLim/LimStat_f32  RequirementInfo="{'linktype_rmi_doors' '0000bb41 (/E-STEER Core/SubSystem Specifications/Application Functions/SF99/SF102A Motor Control Parameter Estimation)' '#SF102A_60' 'true' 'REQ:  SF102A_60' '' ; 'linktype_rmi_doors' '0000bb41 (/E-STEER Core/SubSystem Specifications/Application Functions/SF99/SF102A Motor Control Parameter Estimation)' '#SF102A_77' 'true' 'REQ:  SF102A_77' '' } %GIDa_53c037e7_1e94_4595_8bd4_87398b381b2a"  LoLim=MotCtrlPrmEstimnMotInduDaxLoLim  HiLim=MotCtrlPrmEstimnMotInduDaxHiLim
      settings: AttributesFormatString=|
      | Low Limit: %<LoLim>
      | High Limit:%<HiLim>
  Logical Operator1 : Logic  Operator=OR  AllPortsSameDT=off  OutDataTypeStr=boolean
  Merge : Merge  RequirementInfo={'linktype_rmi_doors' '0000bb41 (/E-STEER Core/SubSystem Specifications/Application Functions/SF99/SF102A Motor Control Parameter Estimation)' '#SF102A_92' 'true' 'REQ:SF102A_92' '' } %GIDa_c01b60de_ddaa_4437_a5e5_2aa6993dab84
  Product : Product  RequirementInfo="{'linktype_rmi_doors' '0000bb41 (/E-STEER Core/SubSystem Specifications/Application Functions/SF99/SF102A Motor Control Parameter Estimation)' '#SF102A_55' 'true' 'REQ:  SF102A_55' '' } %GIDa_41fd7c41_22cc_4c09_8909_2aab87ae8636"
  Q axis Inductance Saturation Scale Factor : BilnrIntrpnCmnX/BilnrIntrpnWithRound_u16_u16CmnXu16MplY  RequirementInfo="{'linktype_rmi_doors' '0000bb41 (/E-STEER Core/SubSystem Specifications/Application Functions/SF99/SF102A Motor Control Parameter Estimation)' '#SF102A_56' 'true' 'REQ:  SF102A_56' '' } %GIDa_c30b1ad5_3674_468d_8413_1c1e4521db86"  XTbl=MotCtrlPrmEstimnMotCurrQaxInduSatnX  MplYTbl=MotCtrlPrmEstimnMotInduDaxSatnScaY  BilnrSelnTbl=MotCtrlPrmEstimnMotCurrDaxInduSatnBilnrSeln
      settings: AttributesFormatString=Bilnr ( u16CmnX , u16MplY )
  MotIndu_Dax_Estimn : Outport  RequirementInfo="{'linktype_rmi_doors' '0000bb41 (/E-STEER Core/SubSystem Specifications/Application Functions/SF99/SF102A Motor Control Parameter Estimation)' '#SF102A_93' 'true' 'REQ:  SF102A_93' '' } %GIDa_c8c066ab_ac4d_413f_9b6c_e33614343aa1"
  MotInduDaxEstimdIvs : Outport  RequirementInfo="{'linktype_rmi_doors' '0000bb41 (/E-STEER Core/SubSystem Specifications/Application Functions/SF99/SF102A Motor Control Parameter Estimation)' '#SF102A_103' 'true' 'REQ:  SF102A_103' '' } %GIDa_42a9a86c_a71e_466e_b117_e6327029dc6e"  Port=2
  wires:
  MotCurr_Abs_Qax/1 -> Q axis Inductance Saturation Scale Factor/1
  MotCurr_Abs_Dax/1 -> Q axis Inductance Saturation Scale Factor/2
  Merge/1 -> Product/1
  Q axis Inductance Saturation Scale Factor/1 -> FixdToFloat_f32_u16/1
  Product/1 -> LimStat_f32/1, Data Store Write/1
  FixdToFloat_f32_u16/1 -> Product/2, Data Store Write1/1
  If/2 -> ElseAction/Action
  If/1 -> IfAction/Action
  ElseAction/1(MotInduDaxNom) -> Merge/2
  IfAction/1(MotInduDaxNom) -> Merge/1
  Logical Operator1/1 -> If/1
  DualEcuFltMtgtnEna/1 -> Logical Operator1/2
  IvtrLoaMtgtnEna/1 -> Logical Operator1/1
  LimStat_f32/1 -> Divide/2, MotIndu_Dax_Estimn/1
  Divide/1 -> LimStat_f1/1
  Constant/1 -> Divide/1
  LimStat_f1/1 -> MotInduDaxEstimdIvs/1

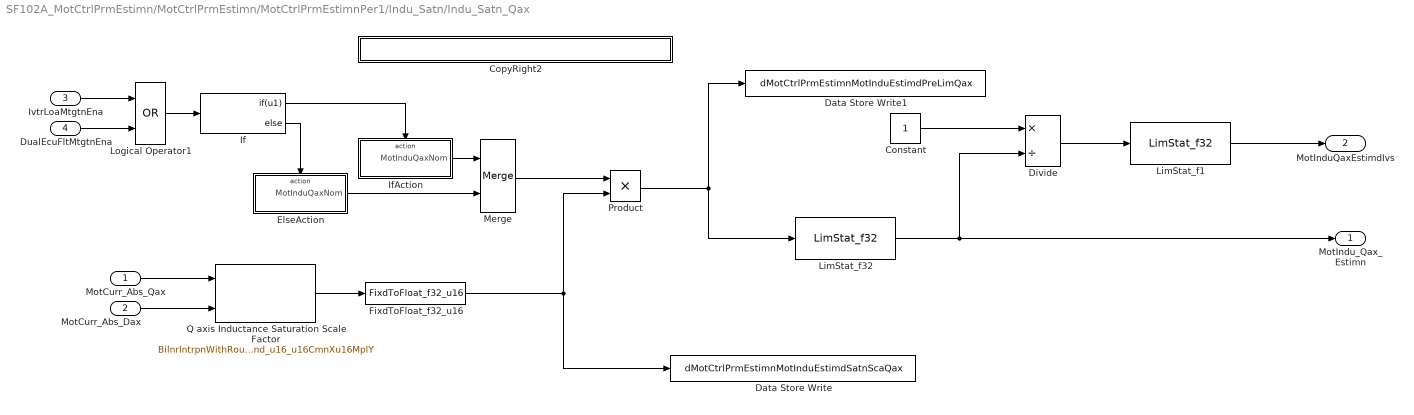
== system SF102A_MotCtrlPrmEstimn/MotCtrlPrmEstimn/MotCtrlPrmEstimnPer1/Indu_Satn/Indu_Satn_Qax ==
  MotCurr_Abs_Qax : Inport  RequirementInfo="{'linktype_rmi_doors' '0000bb41 (/E-STEER Core/SubSystem Specifications/Application Functions/SF99/SF102A Motor Control Parameter Estimation)' '#SF102A_53' 'true' 'REQ:  SF102A_53' '' ; 'linktype_rmi_doors' '0000bb41 (/E-STEER Core/SubSystem Specifications/Application Functions/SF99/SF102A Motor Control Parameter Estimation)' '#SF102A_54' 'true' 'REQ:  SF102A_54' '' } %GIDa_b924f6ea_fc07_44ee_9927_768f35749293"
  MotCurr_Abs_Dax : Inport  RequirementInfo="{'linktype_rmi_doors' '0000bb41 (/E-STEER Core/SubSystem Specifications/Application Functions/SF99/SF102A Motor Control Parameter Estimation)' '#SF102A_53' 'true' 'REQ:  SF102A_53' '' ; 'linktype_rmi_doors' '0000bb41 (/E-STEER Core/SubSystem Specifications/Application Functions/SF99/SF102A Motor Control Parameter Estimation)' '#SF102A_54' 'true' 'REQ:  SF102A_54' '' } %GIDa_06f20df3_3c43_4b7b_9e8d_9aa5cb424bcf"  Port=2
  IvtrLoaMtgtnEna : Inport  RequirementInfo={} %GIDa_1e6c6799_111a_4763_99cd_9bec9441ae05  Port=3
  DualEcuFltMtgtnEna : Inport  RequirementInfo={} %GIDa_04a8051f_c83a_4fc1_942e_952bb1fc2784  Port=4
  Constant : Constant  RequirementInfo={} %GIDa_60957662_8ad2_49b3_abdd_f90055b7125d  OutDataTypeStr=single
  CopyRight2 : Subsystem  Description=|  mask(Copyright Information){none=on}
      | Copyright info block.                                               
      |                                                                     
      | Place copyright information at the top of every subsystem in design.
      mask prompts: none "No parameters"
      mask help: Place copyright information at the top of every subsystem in design.
      mask Display:
      | NxtrConf = 'Nexteer Confidential';
      | 
      | sys = bdroot; %handle for the current model ("system")
      | first = get_param(sys,'Created');
      | if(isempty(first))
      |     first = datestr(now,'yyyy');
      | else
      |     first = first(end-3:end);  %year is last four digits
      | end
      | 
      | last = get_param(sys,'LastModifiedDate');
      | if isempty(last)
      |     last = datestr(now,'yyyy');
      | else
      |     last = last(end-3:end);
      | end
      | 
      | if strcmp(first,last)
      |     fprintf('%s -- Copyright %s Nexteer',NxtrConf,first)
      | else
      |     fprintf('%s -- %s%s- %s Nexteer',NxtrConf,char(169),first,last)
      | end
  Data Store Write : DataStoreWrite  DataStoreName=dMotCtrlPrmEstimnMotInduEstimdSatnScaQax
  Data Store Write1 : DataStoreWrite  DataStoreName=dMotCtrlPrmEstimnMotInduEstimdPreLimQax
  Divide : Product  Inputs=*/
  ElseAction : Subsystem  RequirementInfo={'linktype_rmi_doors' '0000bb41 (/E-STEER Core/SubSystem Specifications/Application Functions/SF99/SF102A Motor Control Parameter Estimation)' '#SF102A_91' 'true' 'REQ:SF102A_91' '' } %GIDa_bf6ea70f_4955_4032_9701_b825a0f3c414  TreatAsAtomicUnit=on
  FixdToFloat_f32_u16 : FixdToFloat/FixdToFloat_f32_u16  RequirementInfo="{'linktype_rmi_doors' '0000bb41 (/E-STEER Core/SubSystem Specifications/Application Functions/SF99/SF102A Motor Control Parameter Estimation)' '#SF102A_53' 'true' 'REQ:  SF102A_53' '' } %GIDa_0c5924cd_57ac_4616_a672_4692d7299331"  Param1=14
  If : If  RequirementInfo={'linktype_rmi_doors' '0000bb41 (/E-STEER Core/SubSystem Specifications/Application Functions/SF99/SF102A Motor Control Parameter Estimation)' '#SF102A_91' 'true' 'REQ:SF102A_91' '' } %GIDa_29f27ca3_0e2d_4334_8211_d6bb189ffc04  IfExpression=u1
  IfAction : Subsystem  RequirementInfo={'linktype_rmi_doors' '0000bb41 (/E-STEER Core/SubSystem Specifications/Application Functions/SF99/SF102A Motor Control Parameter Estimation)' '#SF102A_91' 'true' 'REQ:SF102A_91' '' } %GIDa_a6823c2f_a1c9_4c76_bb3f_f907a2de91f0  TreatAsAtomicUnit=on
      settings: RTWSystemCode=Inline
  LimStat_f1 : NxtrLim/LimStat_f32  RequirementInfo="{'linktype_rmi_doors' '0000bb41 (/E-STEER Core/SubSystem Specifications/Application Functions/SF99/SF102A Motor Control Parameter Estimation)' '#SF102A_77' 'true' 'REQ:  SF102A_77' '' } %GIDa_ee03d579_13fc_4fe8_a93a_6cac7f5e05a8"  LoLim=MOTINDUIVSLOLIM_IVSHENRY_F32  HiLim=MOTINDUIVSHILIM_IVSHENRY_F32
      settings: AttributesFormatString=|
      | Low Limit: %<LoLim>
      | High Limit:%<HiLim>
  LimStat_f32 : NxtrLim/LimStat_f32  RequirementInfo="{'linktype_rmi_doors' '0000bb41 (/E-STEER Core/SubSystem Specifications/Application Functions/SF99/SF102A Motor Control Parameter Estimation)' '#SF102A_60' 'true' 'REQ:  SF102A_60' '' ; 'linktype_rmi_doors' '0000bb41 (/E-STEER Core/SubSystem Specifications/Application Functions/SF99/SF102A Motor Control Parameter Estimation)' '#SF102A_77' 'true' 'REQ:  SF102A_77' '' } %GIDa_883b457e_b373_41e6_8ca5_b830e4b4d362"  LoLim=MotCtrlPrmEstimnMotInduQaxLoLim  HiLim=MotCtrlPrmEstimnMotInduQaxHiLim
      settings: AttributesFormatString=|
      | Low Limit: %<LoLim>
      | High Limit:%<HiLim>
  Logical Operator1 : Logic  Operator=OR  AllPortsSameDT=off  OutDataTypeStr=boolean
  Merge : Merge  RequirementInfo={'linktype_rmi_doors' '0000bb41 (/E-STEER Core/SubSystem Specifications/Application Functions/SF99/SF102A Motor Control Parameter Estimation)' '#SF102A_91' 'true' 'REQ:SF102A_91' '' } %GIDa_3cb74d31_eb79_4be4_8dc6_53ddc180b324
  Product : Product  RequirementInfo={'linktype_rmi_doors' '0000bb41 (/E-STEER Core/SubSystem Specifications/Application Functions/SF99/SF102A Motor Control Parameter Estimation)' '#SF102A_55' 'true' 'REQ:SF102A_55' '' } %GIDa_85a732a5_443c_4bb1_83ab_b5a988731939
  Q axis Inductance Saturation Scale Factor : BilnrIntrpnCmnX/BilnrIntrpnWithRound_u16_u16CmnXu16MplY  RequirementInfo="{'linktype_rmi_doors' '0000bb41 (/E-STEER Core/SubSystem Specifications/Application Functions/SF99/SF102A Motor Control Parameter Estimation)' '#SF102A_53' 'true' 'REQ:  SF102A_53' '' } %GIDa_b6c19266_5888_4c20_a5b2_121b0b219822"  XTbl=MotCtrlPrmEstimnMotCurrQaxInduSatnX  MplYTbl=MotCtrlPrmEstimnMotInduQaxSatnScaY  BilnrSelnTbl=MotCtrlPrmEstimnMotCurrDaxInduSatnBilnrSeln
      settings: AttributesFormatString=Bilnr ( u16CmnX , u16MplY )
  MotIndu_Qax_Estimn : Outport  RequirementInfo="{'linktype_rmi_doors' '0000bb41 (/E-STEER Core/SubSystem Specifications/Application Functions/SF99/SF102A Motor Control Parameter Estimation)' '#SF102A_55' 'true' 'REQ:  SF102A_55' '' } %GIDa_2ed5a014_39f7_4426_89d1_de00eec0cb90"
  MotInduQaxEstimdIvs : Outport  RequirementInfo="{'linktype_rmi_doors' '0000bb41 (/E-STEER Core/SubSystem Specifications/Application Functions/SF99/SF102A Motor Control Parameter Estimation)' '#SF102A_102' 'true' 'REQ:  SF102A_102' '' } %GIDa_6e30658f_e1ae_4a2a_9bc9_9e8ced7b51af"  Port=2
  wires:
  MotCurr_Abs_Qax/1 -> Q axis Inductance Saturation Scale Factor/1
  MotCurr_Abs_Dax/1 -> Q axis Inductance Saturation Scale Factor/2
  Merge/1 -> Product/1
  Q axis Inductance Saturation Scale Factor/1 -> FixdToFloat_f32_u16/1
  Product/1 -> LimStat_f32/1, Data Store Write1/1
  FixdToFloat_f32_u16/1 -> Product/2, Data Store Write/1
  If/2 -> ElseAction/Action
  If/1 -> IfAction/Action
  ElseAction/1(MotInduQaxNom) -> Merge/2
  IfAction/1(MotInduQaxNom) -> Merge/1
  Logical Operator1/1 -> If/1
  IvtrLoaMtgtnEna/1 -> Logical Operator1/1
  DualEcuFltMtgtnEna/1 -> Logical Operator1/2
  LimStat_f32/1 -> Divide/2, MotIndu_Qax_Estimn/1
  Divide/1 -> LimStat_f1/1
  Constant/1 -> Divide/1
  LimStat_f1/1 -> MotInduQaxEstimdIvs/1

== system SF102A_MotCtrlPrmEstimn/MotCtrlPrmEstimn/MotCtrlPrmEstimnPer1/Ke_Satn/CopyRight2 ==

== system SF102A_MotCtrlPrmEstimn/MotCtrlPrmEstimn/MotCtrlPrmEstimnPer1/Ke_Satn/ElseAction ==
  MotKeSatSca : Inport  RequirementInfo={} %GIDa_5c713fa5_7d27_425f_a800_64164b87e56e
  Action Port : ActionPort  ActionType=else
  MotKeSatScaAdj : Outport
  wires:
  MotKeSatSca/1 -> MotKeSatScaAdj/1

== system SF102A_MotCtrlPrmEstimn/MotCtrlPrmEstimn/MotCtrlPrmEstimnPer1/Ke_Satn/IfAction ==
  MotKeSatSca : Inport  RequirementInfo={} %GIDa_6eff96e5_8bfc_4afd_b562_5743b0c1fcd7
  Action Port : ActionPort  ActionType=then
  Add : Sum  Inputs=+-
  Add1 : Sum  Inputs=+-
  Constant : Constant  RequirementInfo={} %GIDa_6fa121bc_1442_4761_a9df_bf797725a658  OutDataTypeStr=single
  Constant1 : Constant  RequirementInfo={'linktype_rmi_doors' '0000bb41 (/E-STEER Core/SubSystem Specifications/Application Functions/SF99/SF102A Motor Control Parameter Estimation)' '#SF102A_97' 'true' 'REQ:SF102A_97' '' } %GIDa_f6db8b21_b160_48e6_9e7b_f0dce4279684  Value=MotCtrlPrmEstimnMotBackEmfConSatnScaIvtrLoaMtgtn
  Constant2 : Constant  RequirementInfo={} %GIDa_030dccf9_416a_4b10_9a2e_e5d5876a0b04  OutDataTypeStr=single
  Product : Product  RequirementInfo={} %GIDa_52e661ea_78ab_4621_9fd9_eb90b6dfc9fd
  MotKeSatScaAdj : Outport
  wires:
  Constant/1 -> Add/1
  MotKeSatSca/1 -> Add/2
  Add/1 -> Product/1
  Constant1/1 -> Product/2
  Constant2/1 -> Add1/1
  Product/1 -> Add1/2
  Add1/1 -> MotKeSatScaAdj/1

== system SF102A_MotCtrlPrmEstimn/MotCtrlPrmEstimn/MotCtrlPrmEstimnPer2/Estimate_Motor_Ke/CopyRight2 ==

== system SF102A_MotCtrlPrmEstimn/MotCtrlPrmEstimn/MotCtrlPrmEstimnPer2/Estimate_Motor_Resitance/CopyRight2 ==

== system SF102A_MotCtrlPrmEstimn/MotCtrlPrmEstimn/MotCtrlPrmEstimnPer1/Indu_Satn/Indu_Satn_Dax/CopyRight2 ==

== system SF102A_MotCtrlPrmEstimn/MotCtrlPrmEstimn/MotCtrlPrmEstimnPer1/Indu_Satn/Indu_Satn_Dax/ElseAction ==
  Action Port : ActionPort  ActionType=else
  Constant : Constant  RequirementInfo={'linktype_rmi_doors' '0000bb41 (/E-STEER Core/SubSystem Specifications/Application Functions/SF99/SF102A Motor Control Parameter Estimation)' '#SF102A_90' 'true' 'REQ:SF102A_90' '' } %GIDa_d86fa906_841d_4403_b05e_6156025ff8df  Value=MotCtrlPrmEstimnMotInduDaxNom
  MotInduDaxNom : Outport
  wires:
  Constant/1 -> MotInduDaxNom/1

== system SF102A_MotCtrlPrmEstimn/MotCtrlPrmEstimn/MotCtrlPrmEstimnPer1/Indu_Satn/Indu_Satn_Dax/IfAction ==
  Action Port : ActionPort  ActionType=then
  Constant : Constant  RequirementInfo="{'linktype_rmi_doors' '0000bb41 (/E-STEER Core/SubSystem Specifications/Application Functions/SF99/SF102A Motor Control Parameter Estimation)' '#SF102A_105' 'true' 'REQ:  SF102A_105' '' } %GIDa_11614c90_8caf_46a4_9b75_8799e2993877"  Value=MotCtrlPrmEstimnMotInduDaxIvtrLoaMtgtn
  MotInduDaxNom : Outport
  wires:
  Constant/1 -> MotInduDaxNom/1

== system SF102A_MotCtrlPrmEstimn/MotCtrlPrmEstimn/MotCtrlPrmEstimnPer1/Indu_Satn/Indu_Satn_Qax/CopyRight2 ==

== system SF102A_MotCtrlPrmEstimn/MotCtrlPrmEstimn/MotCtrlPrmEstimnPer1/Indu_Satn/Indu_Satn_Qax/ElseAction ==
  Action Port : ActionPort  ActionType=else
  Constant : Constant  RequirementInfo={'linktype_rmi_doors' '0000bb41 (/E-STEER Core/SubSystem Specifications/Application Functions/SF99/SF102A Motor Control Parameter Estimation)' '#SF102A_89' 'true' 'REQ:SF102A_89' '' } %GIDa_43c6cdc7_d405_4a71_b78e_8ca386385037  Value=MotCtrlPrmEstimnMotInduQaxNom
  MotInduQaxNom : Outport
  wires:
  Constant/1 -> MotInduQaxNom/1

== system SF102A_MotCtrlPrmEstimn/MotCtrlPrmEstimn/MotCtrlPrmEstimnPer1/Indu_Satn/Indu_Satn_Qax/IfAction ==
  Action Port : ActionPort  ActionType=then
  Constant : Constant  RequirementInfo="{'linktype_rmi_doors' '0000bb41 (/E-STEER Core/SubSystem Specifications/Application Functions/SF99/SF102A Motor Control Parameter Estimation)' '#SF102A_104' 'true' 'REQ:  SF102A_104' '' } %GIDa_afa5a0d7_11aa_4c05_affc_166e7b75013c"  Value=MotCtrlPrmEstimnMotInduQaxIvtrLoaMtgtn
  MotInduQaxNom : Outport
  wires:
  Constant/1 -> MotInduQaxNom/1
